simulink model "RC_3L_PWM"  (R2013b)
settings: Solver=FixedStepDiscrete  SolverMode=SingleTasking  StartTime=0.0  StopTime=1  FixedStep=Tpas  RelTol=1e-3
undefined symbols (not defined in the file): Cbus, fmod4Q, Freq, IAFE3L, IDCP, Kac, Lac, PAFE3L, PDCP, Rac, Rch, Satv, Tpas, Vac, Vdc
libraries: powerlib x39, simulink x33, powerlib_meascontrol x11
settings Model: Creator=LiberT  LastModifiedBy=LiberT
settings DataIOCC: SignalLoggingSaveFormat=ModelDataLogs
settings OptimizationCC: ExpressionDepthLimit=2147483647
settings DebuggingCC: MultiTaskDSMMsg=warning  MultiTaskCondExecSysMsg=none  FcnCallInpInsideContextMsg=EnableAllAsWarning  StateNameClashWarn=warning
settings RTWCC: IncludeERTFirstTime=on

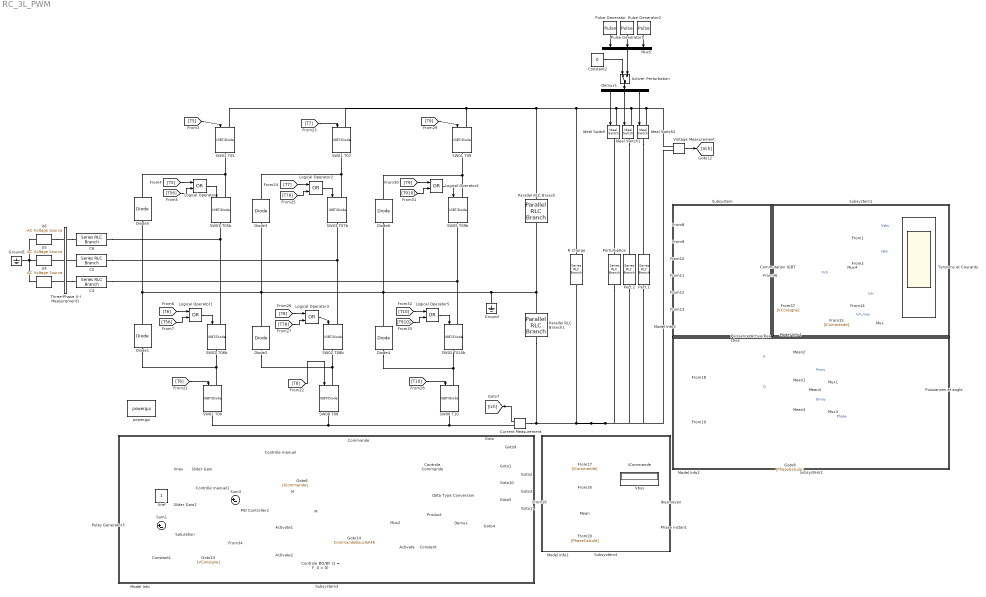
== system RC_3L_PWM ==
  " Controle BO/BF (1 = F, 0 = 0)" : ManualSwitch
  Activate : Constant  Value=0  SampleTime=Tpas
  Activate1 : Constant  SampleTime=Tpas
  Activate2 : Constant  Value=0  SampleTime=Tpas
  Activer Perturbation : ManualSwitch
  C4 : powerlib/Elements/Series RLC Branch  LConnTagsString=__new0  RConnTagsString=__new0  BranchType=L  Resistance=Rac  Inductance=Lac  SetiL0=off  InitialCurrent=0  Capacitance=300e-3  Setx0=off  InitialVoltage=0  Measurements=None
  C5 : powerlib/Elements/Series RLC Branch  LConnTagsString=__new0  RConnTagsString=__new0  BranchType=L  Resistance=Rac  Inductance=Lac  SetiL0=off  InitialCurrent=0  Capacitance=300e-3  Setx0=off  InitialVoltage=0  Measurements=None
  C6 : powerlib/Elements/Series RLC Branch  LConnTagsString=__new0  RConnTagsString=__new0  BranchType=L  Resistance=Rac  Inductance=Lac  SetiL0=off  InitialCurrent=0  Capacitance=300e-3  Setx0=off  InitialVoltage=0  Measurements=None
  Commande : Subsystem
  Commutation IGBT : Scope  NumInputPorts=6
      settings: TickLabels=on  TimeRange=0.002  YMin=-0.2~-0.2~-0.2~-0.2~-0.2~-0.2  YMax=1.2~1.2~1.2~1.2~1.2~1.2
  Constant : Constant  Value=[1 1 1 1 1 1 1 1 1]
  Constant1 : Constant  Value=6000
  Constant2 : Constant  Value=0
  Controle Commande : ManualSwitch
  Contrôle manuel : ManualSwitch  CurrentSetting=0
  Contrôle manuel1 : ManualSwitch  CurrentSetting=0
  Current Measurement : powerlib/Measurements/Current Measurement  PhasorSimulation=off  OutputType=Complex  PSBequivalent=0
  Data Type Conversion : DataTypeConversion  OutDataTypeStr=boolean
  Demux : Demux  Outputs=9
  Demux1 : Demux  Outputs=3
  Diode{1..6} (6 alike) : powerlib/Power Electronics/Diode  Ron=0.001  Lon=0  Vf=0.8  IC=0  UseSnubber=off  Rs=500  Cs=inf  Measurements=off
  Ground : powerlib/Elements/Ground  LConnTagsString=a
  Ground1 : powerlib/Elements/Ground  LConnTagsString=a
  "ICommande " : Display
  Ibusmoyen : Display
  Ideal Switch : powerlib/Power Electronics/Ideal Switch  Ron=0.001  Lon=0  IC=0  Rs=1e5  Cs=inf  Measurements=off
  Ideal Switch1 : powerlib/Power Electronics/Ideal Switch  Ron=0.001  Lon=0  IC=0  Rs=1e5  Cs=inf  Measurements=off
  Ideal Switch2 : powerlib/Power Electronics/Ideal Switch  Ron=0.001  Lon=0  IC=0  Rs=1e5  Cs=inf  Measurements=off
  Imax : Constant  Value=5000
  Logical Operator{,1..5} (6 alike) : Logic  Operator=OR  AllPortsSameDT=off  OutDataTypeStr=boolean
  M : Constant  SampleTime=Tpas
  "M " : simulink/Math Operations/Slider Gain  low=-1  gain=0  high=1
  Mean : powerlib_meascontrol/Measurements/Mean  Freq=50  Vinit=0  Ts=Tpas
  Mean1 : powerlib_meascontrol/Measurements/Mean  Freq=50  Vinit=0  Ts=Tpas
  Mean2 : powerlib_meascontrol/Measurements/Mean  Freq=fmod4Q  Vinit=0  Ts=Tpas
  Mean3 : powerlib_meascontrol/Measurements/Mean  Freq=50  Vinit=0  Ts=Tpas
  Mean4 : powerlib_meascontrol/Measurements/Mean  Freq=fmod4Q  Vinit=0  Ts=Tpas
  Model Info : simulink/Model-Wide Utilities/Model Info  InitialBlockCM=None  BlockCM=None  Frame=on  DisplayStringWithTags=Commande  HorizontalTextAlignment=Center  LeftAlignmentValue=0.5  SourceBlockDiagram=RC_3L_PWM  TagMaxNumber=20
  Model Info{1..4} (4 alike) : simulink/Model-Wide Utilities/Model Info  InitialBlockCM=None  BlockCM=None  Frame=on  DisplayStringWithTags=Résultats  HorizontalTextAlignment=Center  LeftAlignmentValue=0.5  SourceBlockDiagram=RC_3L_PWM  TagMaxNumber=20
  Mux{,1,3..4} (4 alike) : Mux  Inputs=2
  Mux2 : Mux  Inputs=9
  Mux5 : Mux  Inputs=3
  PID Controller2 : simulink/Continuous/PID Controller  Controller=PI  TimeDomain=Discrete-time  SampleTime=Tpas  IntegratorMethod=Forward Euler  FilterMethod=Forward Euler  Form=Parallel  P=PAFE3L  I=IAFE3L  D=0  N=100  InitialConditionSource=internal  InitialConditionForIntegrator=0  InitialConditionForFilter=0  ExternalReset=none  LimitOutput=on  UpperSaturationLimit=Satv  LowerSaturationLimit=-Satv  LinearizeAsGain=on  AntiWindupMode=clamping  Kb=1  TrackingMode=off  Kt=1  PParamMin=[]  PParamMax=[]  IParamMin=[]  IParamMax=[]  DParamMin=[]  DParamMax=[]  NParamMin=[]  NParamMax=[]  KbParamMin=[]  KbParamMax=[]  KtParamMin=[]  KtParamMax=[]  POutMin=[]  POutMax=[]  IOutMin=[]  IOutMax=[]  DOutMin=[]  DOutMax=[]  NOutMin=[]  NOutMax=[]  KbOutMin=[]  KbOutMax=[]  KtOutMin=[]  KtOutMax=[]  IntegratorOutMin=[]  IntegratorOutMax=[]  FilterOutMin=[]  FilterOutMax=[]  SumOutMin=[]  SumOutMax=[]  SumI1OutMin=[]  SumI1OutMax=[]  SumI2OutMin=[]  SumI2OutMax=[]  SumI3OutMin=[]  SumI3OutMax=[]  SumDOutMin=[]  SumDOutMax=[]  SaturationOutMin=[]  SaturationOutMax=[]  IntegratorContinuousStateAttributes=''  IntegratorStateMustResolveToSignalObject=off  IntegratorRTWStateStorageClass=Auto  FilterContinuousStateAttributes=''  FilterStateMustResolveToSignalObject=off  FilterRTWStateStorageClass=Auto
  Parallel RLC Branch : powerlib/Elements/Parallel RLC Branch  LConnTagsString=a  RConnTagsString=__new0  BranchType=C  Resistance=9.26  Inductance=1e-3  SetiL0=off  InitialCurrent=0  Capacitance=Cbus*2  Setx0=on  InitialVoltage=Vdc/2  Measurements=None
  Parallel RLC Branch1 : powerlib/Elements/Parallel RLC Branch  LConnTagsString=a  RConnTagsString=__new0  BranchType=C  Resistance=9.26  Inductance=1e-3  SetiL0=off  InitialCurrent=0  Capacitance=Cbus*2  Setx0=on  InitialVoltage=Vdc/2  Measurements=None
  Pert.1 : powerlib/Elements/Series RLC Branch  LConnTagsString=__new0  RConnTagsString=__new0  BranchType=R  Resistance=50  Inductance=0  SetiL0=off  InitialCurrent=0  Capacitance=inf  Setx0=off  InitialVoltage=0  Measurements=None
  Pert.2 : powerlib/Elements/Series RLC Branch  LConnTagsString=__new0  RConnTagsString=__new0  BranchType=R  Resistance=50  Inductance=0  SetiL0=off  InitialCurrent=0  Capacitance=inf  Setx0=off  InitialVoltage=0  Measurements=None
  Perturbation : powerlib/Elements/Series RLC Branch  LConnTagsString=__new0  RConnTagsString=__new0  BranchType=R  Resistance=50  Inductance=0  SetiL0=off  InitialCurrent=0  Capacitance=inf  Setx0=off  InitialVoltage=0  Measurements=None
  Phase instant. : Display
  Product : Product
  Puissance Active/Reactive : Subsystem
  Puissances et angle : Scope  NumInputPorts=3
      settings: TickLabels=on  TimeRange=0.04  YMin=-5.5e+06~-500000~-120  YMax=500000~250000~50  SaveName=ScopeData2
  Pulse Generator : DiscretePulseGenerator  Period=floor((1/Tpas)/2)  PulseWidth=floor((1/Tpas)/4)  SampleTime=Tpas
  Pulse Generator1 : DiscretePulseGenerator  Period=floor((1/Tpas)/3)  PulseWidth=floor((1/Tpas)/6)  SampleTime=Tpas
  Pulse Generator2 : DiscretePulseGenerator  Period=floor((1/Tpas))  PulseWidth=floor((1/Tpas)/2)  SampleTime=Tpas
  Pulse Generator3 : DiscretePulseGenerator  Amplitude=12000  Period=floor(.4/Tpas)  PulseWidth=floor(.4/2/Tpas)  SampleTime=Tpas
  R Charge : powerlib/Elements/Series RLC Branch  LConnTagsString=__new0  RConnTagsString=__new0  BranchType=R  Resistance=Rch  Inductance=0  SetiL0=off  InitialCurrent=0  Capacitance=inf  Setx0=off  InitialVoltage=0  Measurements=None
  SW01 T05 : powerlib/Power Electronics/IGBT//Diode  Ron=1e-3  Rs=1e5  Cs=Tpas  Measurements=off
  SW01 T05b : powerlib/Power Electronics/IGBT//Diode  Ron=1e-3  Rs=1e5  Cs=Tpas  Measurements=off
  SW01 T07 : powerlib/Power Electronics/IGBT//Diode  Ron=1e-3  Rs=1e5  Cs=Tpas  Measurements=off
  SW01 T09 : powerlib/Power Electronics/IGBT//Diode  Ron=1e-3  Rs=1e5  Cs=Tpas  Measurements=off
  SW02 T010b : powerlib/Power Electronics/IGBT//Diode  Ron=1e-3  Rs=1e5  Cs=Tpas  Measurements=off
  SW02 T06 : powerlib/Power Electronics/IGBT//Diode  Ron=1e-3  Rs=1e5  Cs=Tpas  Measurements=off
  SW02 T06b : powerlib/Power Electronics/IGBT//Diode  Ron=1e-3  Rs=1e5  Cs=Tpas  Measurements=off
  SW02 T08b : powerlib/Power Electronics/IGBT//Diode  Ron=1e-3  Rs=1e5  Cs=Tpas  Measurements=off
  SW03 T07b : powerlib/Power Electronics/IGBT//Diode  Ron=1e-3  Rs=1e5  Cs=Tpas  Measurements=off
  SW04 T08 : powerlib/Power Electronics/IGBT//Diode  Ron=1e-3  Rs=1e5  Cs=Tpas  Measurements=off
  SW05 T09b : powerlib/Power Electronics/IGBT//Diode  Ron=1e-3  Rs=1e5  Cs=Tpas  Measurements=off
  SW06 T10 : powerlib/Power Electronics/IGBT//Diode  Ron=1e-3  Rs=1e5  Cs=Tpas  Measurements=off
  Saturation : Saturate  UpperLimit=5100  LowerLimit=5000
  Slider Gain : simulink/Math Operations/Slider Gain  low=0  gain=0.3  high=1
  Slider Gain2 : simulink/Math Operations/Slider Gain  low=0  gain=5000  high=6000
  Subsystem : Subsystem
      mask Display: disp('')
  Subsystem1 : Subsystem
      mask Display: disp('')
  Subsystem2 : Subsystem
      mask Display: disp('')
  Subsystem3 : Subsystem
      mask Display: disp('')
  Subsystem4 : Subsystem
      mask Display: disp('')
  Sum1 : Sum  Inputs=|+-
  Sum3 : Sum  Inputs=|+-
  Tensions et Courants : Scope  NumInputPorts=4
      settings: TickLabels=on  ShowLegends=on  TimeRange=0.4  YMin=-2000~-3000~5000~-1000  YMax=2000~3000~5200~3000  MaxDataPoints=50000
  Three-Phase V-I Measurement1 : powerlib/Measurements/Three-Phase V-I Measurement  VoltageMeasurement=phase-to-ground  SetLabelV=on  LabelV=Vabc  Vpu=off  VpuLL=off  CurrentMeasurement=yes  SetLabelI=on  LabelI=Iabc  Ipu=off  Pbase=100e6  Vbase=500e3  OutputType=Complex  PhasorSimulation=off  PSBequivalent=0
  U4 : powerlib/Electrical Sources/AC Voltage Source  Amplitude=Vac*sqrt(2/3)  Phase=120  Frequency=Freq  SampleTime=Tpas  Measurements=Voltage
  U5 : powerlib/Electrical Sources/AC Voltage Source  Amplitude=Vac*sqrt(2/3)  Phase=-120  Frequency=Freq  SampleTime=Tpas  Measurements=Voltage
  U6 : powerlib/Electrical Sources/AC Voltage Source  Amplitude=Vac*sqrt(2/3)  Phase=0  Frequency=Freq  SampleTime=Tpas  Measurements=Voltage
  Vbus : Display
  Voltage Measurement : powerlib/Measurements/Voltage Measurement  PhasorSimulation=off  OutputType=Complex  PSBequivalent=0
  Vref : Constant  SampleTime=Tpas
  powergui : powerlib/powergui  Priority=1  SimulationMode=Discrete  SolverType=Tustin  SampleTime=Tpas  frequency=60  SPID=off  DisableSnubberDevices=off  DisableRonSwitches=off  DisableVfSwitches=off  SwTol=0  Interpol=off  DisplayEquations=off  frequencyindice=50  Pbase=100e6  ErrMax=1e-4  Iterations=50  UnitsV=kV  UnitsW=MW  FunctionMessages=off  echomessages=off  HookPort=off  EnableUseOfTLC=off  x0status=blocks  RestoreLinks=warning  ResistiveCurrentMeasurement=off  Frange=[0:2:500]  Ylog=off  Xlog=on  ShowGrid=off  save=off  variable=ZData  structure=ScopeData  ZoomFFT=off  StartTime=0.25  cycles=4  DisplayStyle=1  fundamental=50  FreqAxis=off  MaxFrequency=5000  frequencyindicesteady=1  RmsSteady=1  display=off  Ts=0  methode=off
  tag scope: CommandeBoucleAFE=global
  wires:
  Current Measurement/1 -> [Ich]
  [T5] -> Commutation IGBT/1
  [T6] -> Commutation IGBT/2
  [T7] -> Commutation IGBT/3
  [T8] -> Commutation IGBT/4
  [T9] -> Commutation IGBT/5
  [T10] -> Commutation IGBT/6
  [Vabc] -> Tensions et Courants/1  "Vabc"
  [Iabc] -> Tensions et Courants/2  "Iabc"
  Imax/1 -> Slider Gain/1
  [Ich] -> Mux/1  "Ich"
  [ICommande] -> Mux/2  "Ich_moy"
  Mux/1 -> Tensions et Courants/4
  Mean/1 -> Ibusmoyen/1
  [Vch] -> Vbus/1
  [Ich] -> Mean/1
  [ICommande] -> "ICommande "/1
  [Vch] -> Sum3/2
  Vref/1 -> Slider Gain2/1
  Constant/1 -> Product/2
  Activate/1 -> Product/1
  Controle Commande/1 -> Demux/1
  Mux2/1 -> Controle Commande/1
  [Vabc] -> Puissance Active/Reactive/1(Vabc)
  [Iabc] -> Puissance Active/Reactive/2(Iabc)
  Puissance Active/Reactive/1(P) -> Mean2/1, Mean1/1  "P"
  Puissance Active/Reactive/2(Q) -> Mean3/1, Mean4/1  "Q"
  Puissance Active/Reactive/3(PhC) -> Puissances et angle/3, [PhaseCalcule]  "Phase"
  Mean1/1 -> Mux1/2  "Pmoy"
  Mux1/1 -> Puissances et angle/1
  Mean3/1 -> Mux3/2  "Qmoy"
  Mux3/1 -> Puissances et angle/2
  Mux4/1 -> Tensions et Courants/3
  [Vch] -> Mux4/1  "Vch"
  Demux1/1 -> Ideal Switch/1
  Demux1/2 -> Ideal Switch1/1
  Demux1/3 -> Ideal Switch2/1
  Pulse Generator/1 -> Mux5/1
  Pulse Generator1/1 -> Mux5/2
  Pulse Generator2/1 -> Mux5/3
  Activer Perturbation/1 -> Demux1/1
  Mux5/1 -> Activer Perturbation/2
  [PhaseCalcule] -> Phase instant./1
  Sum3/1 -> PID Controller2/1
  Slider Gain/1 -> Contrôle manuel/1
  Contrôle manuel/1 -> Commande/1(In1), [ICommande]
  Data Type Conversion/1 -> Controle Commande/2
  Product/1 -> Data Type Conversion/1
  Sum1/1 -> Saturation/1
  Pulse Generator3/1 -> Sum1/1
  Constant1/1 -> Sum1/2
  Contrôle manuel1/1 -> [VConsigne], Sum3/1
  Slider Gain2/1 -> Contrôle manuel1/1
  Saturation/1 -> Contrôle manuel1/2
  Commande/1(T5) -> Mux2/1
  Commande/2(T56) -> Mux2/2
  Commande/3(T6) -> Mux2/3
  Commande/4(T7) -> Mux2/4
  Commande/5(T78) -> Mux2/5
  Commande/6(T8) -> Mux2/6
  Commande/7(T9) -> Mux2/7
  Commande/8(T89) -> Mux2/8
  Commande/9(T10) -> Mux2/9
  Demux/1 -> [T5]
  Demux/3 -> [T6]
  Demux/4 -> [T7]
  Demux/6 -> [T8]
  Demux/7 -> [T9]
  Demux/9 -> [T10]
  Demux/2 -> [T56]
  Demux/5 -> [T78]
  Demux/8 -> [T910]
  [T5] -> SW01 T05/1
  Logical Operator/1 -> SW01 T05b/1
  [T5] -> Logical Operator/1
  [T56] -> Logical Operator/2
  Logical Operator1/1 -> SW02 T06b/1
  [T6] -> Logical Operator1/1
  [T56] -> Logical Operator1/2
  [T6] -> SW02 T06/1
  [T7] -> SW01 T07/1
  Logical Operator2/1 -> SW03 T07b/1
  [T7] -> Logical Operator2/1
  [T78] -> Logical Operator2/2
  Logical Operator3/1 -> SW02 T08b/1
  [T8] -> Logical Operator3/1
  [T78] -> Logical Operator3/2
  [T8] -> SW04 T08/1
  [T9] -> SW01 T09/1
  Logical Operator4/1 -> SW05 T09b/1
  [T9] -> Logical Operator4/1
  [T910] -> Logical Operator4/2
  Logical Operator5/1 -> SW02 T010b/1
  [T10] -> Logical Operator5/1
  [T910] -> Logical Operator5/2
  [T10] -> SW06 T10/1
  Voltage Measurement/1 -> [Vch]
  Constant2/1 -> Activer Perturbation/1
  [VConsigne] -> Mux4/2
  PID Controller2/1 -> Contrôle manuel/2
  Mean2/1 -> Mux1/1
  Mean4/1 -> Mux3/1
  Activate1/1 -> " Controle BO/BF (1 = F, 0 = 0)"/1
  Activate2/1 -> " Controle BO/BF (1 = F, 0 = 0)"/2
  " Controle BO/BF (1 = F, 0 = 0)"/1 -> [CommandeBoucleAFE]
  "M "/1 -> Commande/2(M)
  M/1 -> "M "/1
  connections:
  SW02 T06b/LConn1 -- SW01 T05b/RConn1 -- C6/LConn1
  SW02 T010b/LConn1 -- C4/LConn1 -- SW05 T09b/RConn1
  SW02 T08b/LConn1 -- C5/LConn1 -- SW03 T07b/RConn1
  Current Measurement/LConn1 -- Voltage Measurement/LConn2 -- Pert.1/RConn1 -- Pert.2/RConn1 -- Perturbation/RConn1 -- R Charge/RConn1 -- Parallel RLC Branch1/RConn1
  Ideal Switch1/RConn1 -- Pert.2/LConn1
  Ideal Switch2/RConn1 -- Pert.1/LConn1
  SW01 T05b/LConn1 -- Diode5/RConn1 -- SW01 T05/RConn1
  SW03 T07b/LConn1 -- Diode3/RConn1 -- SW01 T07/RConn1
  SW05 T09b/LConn1 -- Diode6/RConn1 -- SW01 T09/RConn1
  SW02 T06b/RConn1 -- Diode1/LConn1 -- SW02 T06/LConn1
  SW02 T010b/RConn1 -- Diode4/LConn1 -- SW06 T10/LConn1
  SW04 T08/LConn1 -- Diode2/LConn1 -- SW02 T08b/RConn1
  SW02 T06/RConn1 -- SW06 T10/RConn1 -- Current Measurement/RConn1 -- SW04 T08/RConn1
  SW01 T05/LConn1 -- SW01 T07/LConn1 -- SW01 T09/LConn1 -- Voltage Measurement/LConn1 -- Ideal Switch2/LConn1 -- Ideal Switch1/LConn1 -- Ideal Switch/LConn1 -- R Charge/LConn1 -- Parallel RLC Branch/LConn1
  Diode4/RConn1 -- Diode6/LConn1 -- Ground/LConn1 -- Parallel RLC Branch/RConn1 -- Parallel RLC Branch1/LConn1 -- Diode3/LConn1 -- Diode2/RConn1 -- Diode5/LConn1 -- Diode1/RConn1
  Three-Phase V-I Measurement1/RConn2 -- U5/RConn1
  Three-Phase V-I Measurement1/LConn1 -- C6/RConn1
  C5/RConn1 -- Three-Phase V-I Measurement1/LConn2
  Three-Phase V-I Measurement1/LConn3 -- C4/RConn1
  Three-Phase V-I Measurement1/RConn3 -- U4/RConn1
  U6/RConn1 -- Three-Phase V-I Measurement1/RConn1
  Ground1/LConn1 -- U4/LConn1 -- U6/LConn1 -- U5/LConn1
  Perturbation/LConn1 -- Ideal Switch/RConn1

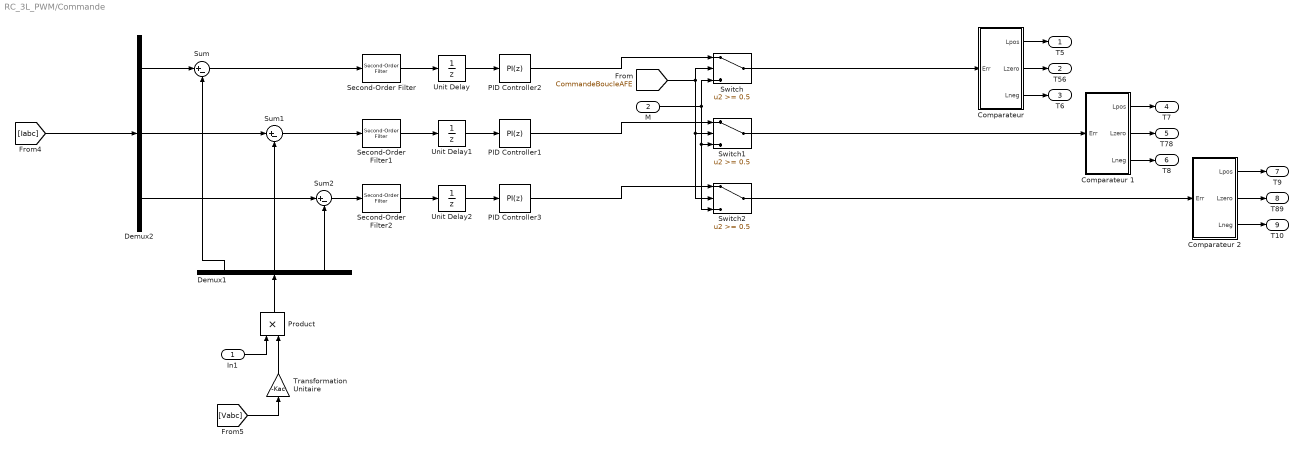
== system RC_3L_PWM/Commande ==
  In1 : Inport
  M : Inport  Port=2
  "Comparateur " : Subsystem
  Comparateur 1 : Subsystem
  Comparateur 2 : Subsystem
  Demux1 : Demux  Outputs=3
  Demux2 : Demux  Outputs=3
  PID Controller1 : simulink/Continuous/PID Controller  Controller=PI  TimeDomain=Discrete-time  SampleTime=Tpas  IntegratorMethod=Forward Euler  FilterMethod=Forward Euler  Form=Parallel  P=PDCP  I=IDCP  D=0  N=100  InitialConditionSource=internal  InitialConditionForIntegrator=0  InitialConditionForFilter=0  ExternalReset=none  LimitOutput=on  UpperSaturationLimit=0.95  LowerSaturationLimit=-0.95  LinearizeAsGain=on  AntiWindupMode=clamping  Kb=1  TrackingMode=off  Kt=1  PParamMin=[]  PParamMax=[]  IParamMin=[]  IParamMax=[]  DParamMin=[]  DParamMax=[]  NParamMin=[]  NParamMax=[]  KbParamMin=[]  KbParamMax=[]  KtParamMin=[]  KtParamMax=[]  POutMin=[]  POutMax=[]  IOutMin=[]  IOutMax=[]  DOutMin=[]  DOutMax=[]  NOutMin=[]  NOutMax=[]  KbOutMin=[]  KbOutMax=[]  KtOutMin=[]  KtOutMax=[]  IntegratorOutMin=[]  IntegratorOutMax=[]  FilterOutMin=[]  FilterOutMax=[]  SumOutMin=[]  SumOutMax=[]  SumI1OutMin=[]  SumI1OutMax=[]  SumI2OutMin=[]  SumI2OutMax=[]  SumI3OutMin=[]  SumI3OutMax=[]  SumDOutMin=[]  SumDOutMax=[]  SaturationOutMin=[]  SaturationOutMax=[]  IntegratorContinuousStateAttributes=''  IntegratorStateMustResolveToSignalObject=off  IntegratorRTWStateStorageClass=Auto  FilterContinuousStateAttributes=''  FilterStateMustResolveToSignalObject=off  FilterRTWStateStorageClass=Auto
  PID Controller2 : simulink/Continuous/PID Controller  Controller=PI  TimeDomain=Discrete-time  SampleTime=Tpas  IntegratorMethod=Forward Euler  FilterMethod=Forward Euler  Form=Parallel  P=PDCP  I=IDCP  D=0  N=100  InitialConditionSource=internal  InitialConditionForIntegrator=0  InitialConditionForFilter=0  ExternalReset=none  LimitOutput=on  UpperSaturationLimit=0.95  LowerSaturationLimit=-0.95  LinearizeAsGain=on  AntiWindupMode=clamping  Kb=1  TrackingMode=off  Kt=1  PParamMin=[]  PParamMax=[]  IParamMin=[]  IParamMax=[]  DParamMin=[]  DParamMax=[]  NParamMin=[]  NParamMax=[]  KbParamMin=[]  KbParamMax=[]  KtParamMin=[]  KtParamMax=[]  POutMin=[]  POutMax=[]  IOutMin=[]  IOutMax=[]  DOutMin=[]  DOutMax=[]  NOutMin=[]  NOutMax=[]  KbOutMin=[]  KbOutMax=[]  KtOutMin=[]  KtOutMax=[]  IntegratorOutMin=[]  IntegratorOutMax=[]  FilterOutMin=[]  FilterOutMax=[]  SumOutMin=[]  SumOutMax=[]  SumI1OutMin=[]  SumI1OutMax=[]  SumI2OutMin=[]  SumI2OutMax=[]  SumI3OutMin=[]  SumI3OutMax=[]  SumDOutMin=[]  SumDOutMax=[]  SaturationOutMin=[]  SaturationOutMax=[]  IntegratorContinuousStateAttributes=''  IntegratorStateMustResolveToSignalObject=off  IntegratorRTWStateStorageClass=Auto  FilterContinuousStateAttributes=''  FilterStateMustResolveToSignalObject=off  FilterRTWStateStorageClass=Auto
  PID Controller3 : simulink/Continuous/PID Controller  Controller=PI  TimeDomain=Discrete-time  SampleTime=Tpas  IntegratorMethod=Forward Euler  FilterMethod=Forward Euler  Form=Parallel  P=PDCP  I=IDCP  D=0  N=100  InitialConditionSource=internal  InitialConditionForIntegrator=0  InitialConditionForFilter=0  ExternalReset=none  LimitOutput=on  UpperSaturationLimit=0.95  LowerSaturationLimit=-0.95  LinearizeAsGain=on  AntiWindupMode=clamping  Kb=1  TrackingMode=off  Kt=1  PParamMin=[]  PParamMax=[]  IParamMin=[]  IParamMax=[]  DParamMin=[]  DParamMax=[]  NParamMin=[]  NParamMax=[]  KbParamMin=[]  KbParamMax=[]  KtParamMin=[]  KtParamMax=[]  POutMin=[]  POutMax=[]  IOutMin=[]  IOutMax=[]  DOutMin=[]  DOutMax=[]  NOutMin=[]  NOutMax=[]  KbOutMin=[]  KbOutMax=[]  KtOutMin=[]  KtOutMax=[]  IntegratorOutMin=[]  IntegratorOutMax=[]  FilterOutMin=[]  FilterOutMax=[]  SumOutMin=[]  SumOutMax=[]  SumI1OutMin=[]  SumI1OutMax=[]  SumI2OutMin=[]  SumI2OutMax=[]  SumI3OutMin=[]  SumI3OutMax=[]  SumDOutMin=[]  SumDOutMax=[]  SaturationOutMin=[]  SaturationOutMax=[]  IntegratorContinuousStateAttributes=''  IntegratorStateMustResolveToSignalObject=off  IntegratorRTWStateStorageClass=Auto  FilterContinuousStateAttributes=''  FilterStateMustResolveToSignalObject=off  FilterRTWStateStorageClass=Auto
  Product : Product
  Second-Order Filter : powerlib_meascontrol/Filters/Second-Order Filter  FilterType=Lowpass  Fo=fmod4Q*1.25  Zeta=0.9  Ts=Tpas  Initialize=on  Vac_Init="[0,  0,  50]"  Vdc_Init=0  PlotResponse=off  FreqRange=[0, 10000, 1]
  Second-Order Filter1 : powerlib_meascontrol/Filters/Second-Order Filter  FilterType=Lowpass  Fo=fmod4Q*1.25  Zeta=0.9  Ts=Tpas  Initialize=on  Vac_Init="[0,  0,  50]"  Vdc_Init=0  PlotResponse=off  FreqRange=[0, 10000, 1]
  Second-Order Filter2 : powerlib_meascontrol/Filters/Second-Order Filter  FilterType=Lowpass  Fo=fmod4Q*1.25  Zeta=0.9  Ts=Tpas  Initialize=on  Vac_Init="[0,  0,  50]"  Vdc_Init=0  PlotResponse=off  FreqRange=[0, 10000, 1]
  Sum : Sum  Inputs=|+-
  Sum1 : Sum  Inputs=|+-
  Sum2 : Sum  Inputs=|+-
  Switch : Switch  Threshold=0.5
  Switch1 : Switch  Threshold=0.5
  Switch2 : Switch  Threshold=0.5
  Transformation Unitaire : Gain  Gain=-Kac
  Unit Delay : UnitDelay  SampleTime=-1
  Unit Delay1 : UnitDelay  SampleTime=-1
  Unit Delay2 : UnitDelay  SampleTime=-1
  T5 : Outport
  T56 : Outport  Port=2
  T6 : Outport  Port=3
  T7 : Outport  Port=4
  T78 : Outport  Port=5
  T8 : Outport  Port=6
  T9 : Outport  Port=7
  T89 : Outport  Port=8
  T10 : Outport  Port=9
  wires:
  Demux2/1 -> Sum/1
  Demux2/2 -> Sum1/1
  Demux2/3 -> Sum2/1
  Unit Delay/1 -> PID Controller2/1
  Unit Delay1/1 -> PID Controller1/1
  Unit Delay2/1 -> PID Controller3/1
  [Vabc] -> Transformation Unitaire/1
  Demux1/1 -> Sum/2
  Demux1/2 -> Sum1/2
  Demux1/3 -> Sum2/2
  Transformation Unitaire/1 -> Product/2
  In1/1 -> Product/1
  Product/1 -> Demux1/1
  "Comparateur "/1(Lpos) -> T5/1
  "Comparateur "/3(Lneg) -> T6/1
  "Comparateur "/2(Lzero) -> T56/1
  Comparateur 1/1(Lpos) -> T7/1
  Comparateur 1/3(Lneg) -> T8/1
  Comparateur 1/2(Lzero) -> T78/1
  Comparateur 2/1(Lpos) -> T9/1
  Comparateur 2/3(Lneg) -> T10/1
  Comparateur 2/2(Lzero) -> T89/1
  [Iabc] -> Demux2/1
  Sum/1 -> Second-Order Filter/1
  Sum1/1 -> Second-Order Filter1/1
  Sum2/1 -> Second-Order Filter2/1
  Second-Order Filter/1 -> Unit Delay/1
  Second-Order Filter1/1 -> Unit Delay1/1
  Second-Order Filter2/1 -> Unit Delay2/1
  PID Controller2/1 -> Switch/1
  Switch/1 -> "Comparateur "/1(Err)
  PID Controller1/1 -> Switch1/1
  Switch1/1 -> Comparateur 1/1(Err)
  PID Controller3/1 -> Switch2/1
  Switch2/1 -> Comparateur 2/1(Err)
  [CommandeBoucleAFE] -> Switch/2, Switch1/2, Switch2/2
  M/1 -> Switch/3, Switch2/3, Switch1/3

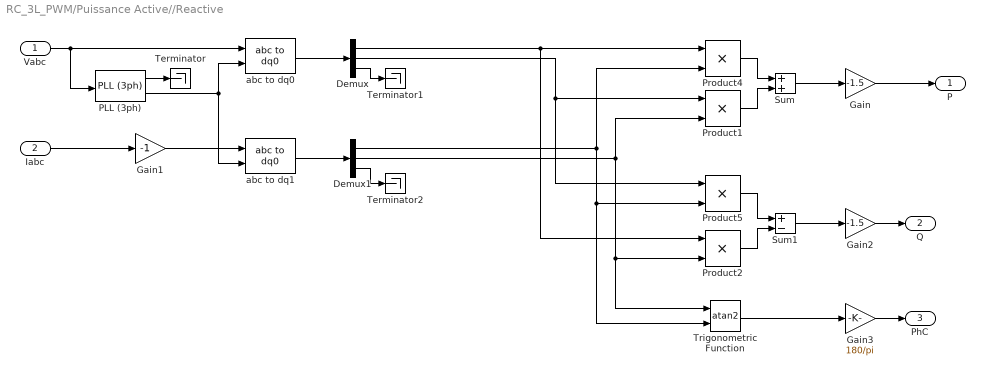
== system RC_3L_PWM/Puissance Active//Reactive ==
  Vabc : Inport
  Iabc : Inport  Port=2
  Demux : Demux  Outputs=3
  Demux1 : Demux  Outputs=3
  Gain : Gain  Gain=-1.5
  Gain1 : Gain  Gain=-1
  Gain2 : Gain  Gain=-1.5
  Gain3 : Gain  Gain=180/pi
  PLL (3ph) : powerlib_meascontrol/PLL/PLL (3ph)  Fmin=49  Par_Init=[0, 50]  ParK=[180, 3200, 1]  TcD=1e-4  MaxRateChangeFreq=6  FilterCutOffFreq=25  Ts=Tpas  AGC=on
  Product{1..2,4..5} (4 alike) : Product
  Sum : Sum
  Sum1 : Sum  Inputs=+-
  Terminator : Terminator
  Terminator1 : Terminator
  Terminator2 : Terminator
  Trigonometric Function : Trigonometry  Operator=atan2
  abc to dq0 : powerlib_meascontrol/Transformations/abc to dq0  Alignment=90 degrees behind phase A axis
  abc to dq1 : powerlib_meascontrol/Transformations/abc to dq0  Alignment=90 degrees behind phase A axis
  P : Outport
  Q : Outport  Port=2
  PhC : Outport  Port=3
  wires:
  Vabc/1 -> PLL (3ph)/1, abc to dq0/1
  abc to dq0/1 -> Demux/1
  abc to dq1/1 -> Demux1/1
  Product2/1 -> Sum1/2
  Sum1/1 -> Gain2/1
  Demux/2 -> Product5/1, Product1/1
  Demux/1 -> Product2/1, Product4/1
  Demux1/2 -> Trigonometric Function/1, Product2/2, Product1/2
  Product5/1 -> Sum1/1
  Gain2/1 -> Q/1
  Trigonometric Function/1 -> Gain3/1
  Gain3/1 -> PhC/1
  Product4/1 -> Sum/1
  Product1/1 -> Sum/2
  Sum/1 -> Gain/1
  Gain/1 -> P/1
  Demux1/1 -> Trigonometric Function/2, Product5/2, Product4/2
  PLL (3ph)/2 -> abc to dq1/2, abc to dq0/2
  Iabc/1 -> Gain1/1
  PLL (3ph)/1 -> Terminator/1
  Demux/3 -> Terminator1/1
  Demux1/3 -> Terminator2/1
  Gain1/1 -> abc to dq1/1

== system RC_3L_PWM/Subsystem ==

== system RC_3L_PWM/Subsystem1 ==

== system RC_3L_PWM/Subsystem2 ==

== system RC_3L_PWM/Subsystem3 ==

== system RC_3L_PWM/Subsystem4 ==

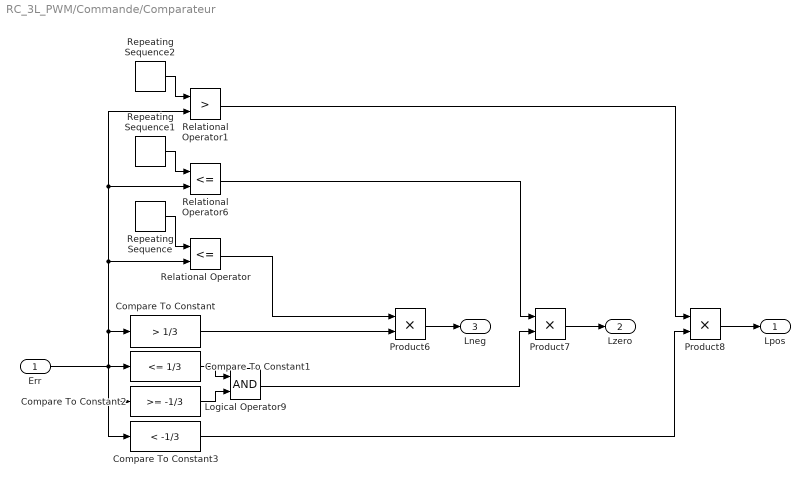
== system RC_3L_PWM/Commande/Comparateur  ==
  Err : Inport
  Compare To Constant : simulink/Logic and Bit Operations/Compare To Constant  relop=>  const=1/3  OutDataTypeStr=boolean
  Compare To Constant1 : simulink/Logic and Bit Operations/Compare To Constant  relop=<=  const=1/3  OutDataTypeStr=boolean
  Compare To Constant2 : simulink/Logic and Bit Operations/Compare To Constant  relop=>=  const=-1/3  OutDataTypeStr=boolean
  Compare To Constant3 : simulink/Logic and Bit Operations/Compare To Constant  relop=<  const=-1/3  OutDataTypeStr=boolean
  Logical Operator9 : Logic  AllPortsSameDT=off  OutDataTypeStr=boolean  SampleTime=Tpas
  Product6 : Product  SampleTime=Tpas
  Product7 : Product  SampleTime=Tpas
  Product8 : Product  SampleTime=Tpas
  Relational Operator : RelationalOperator  Operator=<=  OutDataTypeStr=boolean
  Relational Operator1 : RelationalOperator  Operator=>  OutDataTypeStr=boolean
  Relational Operator6 : RelationalOperator  Operator=<=  OutDataTypeStr=boolean
  Repeating Sequence : simulink/Sources/Repeating Sequence  rep_seq_t=[0 1e-3]  rep_seq_y=[1/3 1.035]
  Repeating Sequence1 : simulink/Sources/Repeating Sequence  rep_seq_t=[0 1e-3]  rep_seq_y=[-.35 .35]
  Repeating Sequence2 : simulink/Sources/Repeating Sequence  rep_seq_t=[0 1e-3]  rep_seq_y=[-1 -1/3]
  Lpos : Outport
  Lzero : Outport  Port=2
  Lneg : Outport  Port=3
  wires:
  Compare To Constant/1 -> Product6/2
  Compare To Constant3/1 -> Product8/2
  Compare To Constant1/1 -> Logical Operator9/1
  Compare To Constant2/1 -> Logical Operator9/2
  Logical Operator9/1 -> Product7/2
  Repeating Sequence/1 -> Relational Operator/1
  Repeating Sequence2/1 -> Relational Operator1/1
  Relational Operator/1 -> Product6/1
  Relational Operator6/1 -> Product7/1
  Relational Operator1/1 -> Product8/1
  Product6/1 -> Lneg/1
  Product8/1 -> Lpos/1
  Product7/1 -> Lzero/1
  Err/1 -> Relational Operator/2, Relational Operator1/2, Relational Operator6/2, Compare To Constant/1, Compare To Constant1/1, Compare To Constant3/1, Compare To Constant2/1
  Repeating Sequence1/1 -> Relational Operator6/1

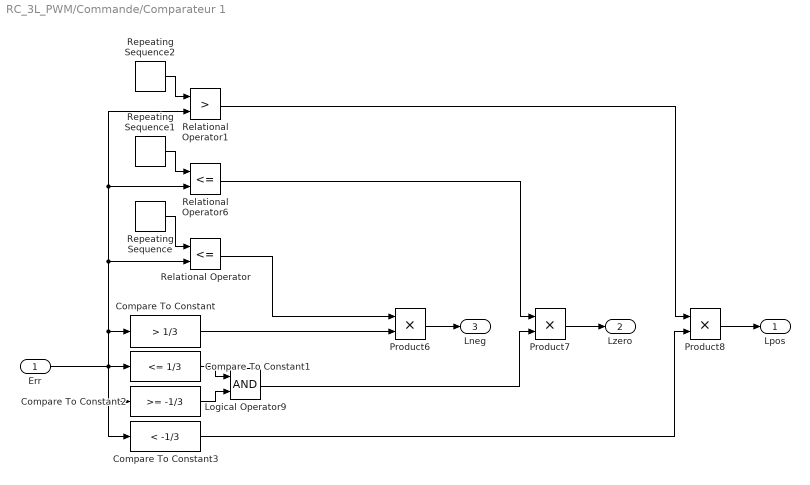
== system RC_3L_PWM/Commande/Comparateur 1 ==
  Err : Inport
  Compare To Constant : simulink/Logic and Bit Operations/Compare To Constant  relop=>  const=1/3  OutDataTypeStr=boolean
  Compare To Constant1 : simulink/Logic and Bit Operations/Compare To Constant  relop=<=  const=1/3  OutDataTypeStr=boolean
  Compare To Constant2 : simulink/Logic and Bit Operations/Compare To Constant  relop=>=  const=-1/3  OutDataTypeStr=boolean
  Compare To Constant3 : simulink/Logic and Bit Operations/Compare To Constant  relop=<  const=-1/3  OutDataTypeStr=boolean
  Logical Operator9 : Logic  AllPortsSameDT=off  OutDataTypeStr=boolean  SampleTime=Tpas
  Product6 : Product  SampleTime=Tpas
  Product7 : Product  SampleTime=Tpas
  Product8 : Product  SampleTime=Tpas
  Relational Operator : RelationalOperator  Operator=<=  OutDataTypeStr=boolean
  Relational Operator1 : RelationalOperator  Operator=>  OutDataTypeStr=boolean
  Relational Operator6 : RelationalOperator  Operator=<=  OutDataTypeStr=boolean
  Repeating Sequence : simulink/Sources/Repeating Sequence  rep_seq_t=[0 1e-3]  rep_seq_y=[1/3 1.035]
  Repeating Sequence1 : simulink/Sources/Repeating Sequence  rep_seq_t=[0 1e-3]  rep_seq_y=[-.35 .35]
  Repeating Sequence2 : simulink/Sources/Repeating Sequence  rep_seq_t=[0 1e-3]  rep_seq_y=[-1 -1/3]
  Lpos : Outport
  Lzero : Outport  Port=2
  Lneg : Outport  Port=3
  wires:
  Compare To Constant/1 -> Product6/2
  Compare To Constant3/1 -> Product8/2
  Compare To Constant1/1 -> Logical Operator9/1
  Compare To Constant2/1 -> Logical Operator9/2
  Logical Operator9/1 -> Product7/2
  Repeating Sequence/1 -> Relational Operator/1
  Repeating Sequence2/1 -> Relational Operator1/1
  Relational Operator/1 -> Product6/1
  Relational Operator6/1 -> Product7/1
  Relational Operator1/1 -> Product8/1
  Product6/1 -> Lneg/1
  Product8/1 -> Lpos/1
  Product7/1 -> Lzero/1
  Err/1 -> Relational Operator/2, Relational Operator1/2, Relational Operator6/2, Compare To Constant/1, Compare To Constant1/1, Compare To Constant3/1, Compare To Constant2/1
  Repeating Sequence1/1 -> Relational Operator6/1

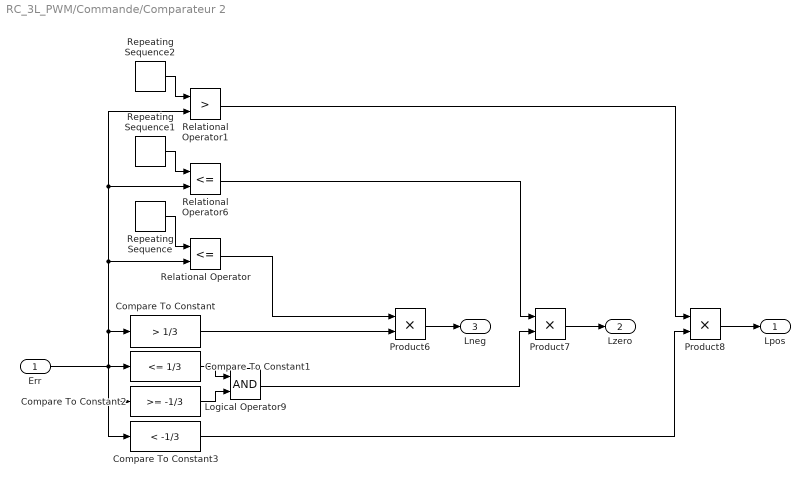
== system RC_3L_PWM/Commande/Comparateur 2 ==
  Err : Inport
  Compare To Constant : simulink/Logic and Bit Operations/Compare To Constant  relop=>  const=1/3  OutDataTypeStr=boolean
  Compare To Constant1 : simulink/Logic and Bit Operations/Compare To Constant  relop=<=  const=1/3  OutDataTypeStr=boolean
  Compare To Constant2 : simulink/Logic and Bit Operations/Compare To Constant  relop=>=  const=-1/3  OutDataTypeStr=boolean
  Compare To Constant3 : simulink/Logic and Bit Operations/Compare To Constant  relop=<  const=-1/3  OutDataTypeStr=boolean
  Logical Operator9 : Logic  AllPortsSameDT=off  OutDataTypeStr=boolean  SampleTime=Tpas
  Product6 : Product  SampleTime=Tpas
  Product7 : Product  SampleTime=Tpas
  Product8 : Product  SampleTime=Tpas
  Relational Operator : RelationalOperator  Operator=<=  OutDataTypeStr=boolean
  Relational Operator1 : RelationalOperator  Operator=>  OutDataTypeStr=boolean
  Relational Operator6 : RelationalOperator  Operator=<=  OutDataTypeStr=boolean
  Repeating Sequence : simulink/Sources/Repeating Sequence  rep_seq_t=[0 1e-3]  rep_seq_y=[1/3 1.035]
  Repeating Sequence1 : simulink/Sources/Repeating Sequence  rep_seq_t=[0 1e-3]  rep_seq_y=[-.35 .35]
  Repeating Sequence2 : simulink/Sources/Repeating Sequence  rep_seq_t=[0 1e-3]  rep_seq_y=[-1 -1/3]
  Lpos : Outport
  Lzero : Outport  Port=2
  Lneg : Outport  Port=3
  wires:
  Compare To Constant/1 -> Product6/2
  Compare To Constant3/1 -> Product8/2
  Compare To Constant1/1 -> Logical Operator9/1
  Compare To Constant2/1 -> Logical Operator9/2
  Logical Operator9/1 -> Product7/2
  Repeating Sequence/1 -> Relational Operator/1
  Repeating Sequence2/1 -> Relational Operator1/1
  Relational Operator/1 -> Product6/1
  Relational Operator6/1 -> Product7/1
  Relational Operator1/1 -> Product8/1
  Product6/1 -> Lneg/1
  Product8/1 -> Lpos/1
  Product7/1 -> Lzero/1
  Err/1 -> Relational Operator/2, Relational Operator1/2, Relational Operator6/2, Compare To Constant/1, Compare To Constant1/1, Compare To Constant3/1, Compare To Constant2/1
  Repeating Sequence1/1 -> Relational Operator6/1
